simulink library "uplink_4c1r_pd_accu_reg_block"  (Simulink 8.7)
settings: Solver=ode45  StartTime=0.0  StopTime=10.0  RelTol=1e-3
undefined symbols (not defined in the file or in its folder): value
libraries: DSPBAPrim x1, Register x1, DSPBABase x1, Accumulator x1, Peak_Detector x1
settings Model: Creator=bigcat  LastModifiedBy=5g

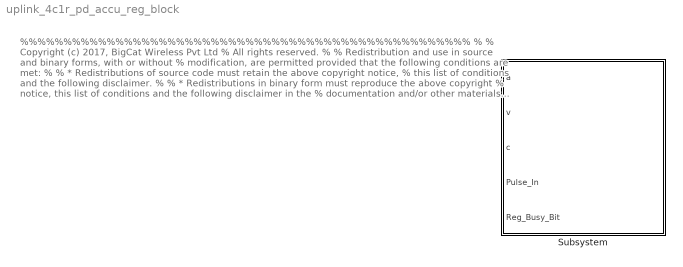
== system uplink_4c1r_pd_accu_reg_block ==
  note: %%%%%%%%%%%%%%%%%%%%%%%%%%%%%%%%%%%%%%%%%%%%%%%%%%%%
      |  %
      |  % Copyright (c) 2017, BigCat Wireless Pvt Ltd
      |  % All rights reserved.
      |  %
      |  % Redistribution and use in source and binary forms, with or without
      |  % modification, are permitted provided that the following conditions are met:
      |  %
      |  %     * Redistributions of source code must retain the above copyright notice,
      |  %       this list of conditions and the following disclaimer.
      |  %
      |  %     * Redistributions in binary form must reproduce the above copyright
      |  %       notice, this list of conditions and the following disclaimer in the
      |  %       documentation and/or other materials provided with the distribution.
      |  %
      |  %     * Neither the name of the copyright holder nor the names of its contributors
      |  %       may be used to endorse or promote products derived from this software
      |  %       without specific prior written permission.
      |  %
      |  %
      |  %
      |  % THIS SOFTWARE IS PROVIDED BY THE COPYRIGHT HOLDERS AND CONTRIBUTORS "AS IS"
      |  % AND ANY EXPRESS OR IMPLIED WARRANTIES, INCLUDING, BUT NOT LIMITED TO, THE
      |  % IMPLIED WARRANTIES OF MERCHANTABILITY AND FITNESS FOR A PARTICULAR PURPOSE ARE
      |  % DISCLAIMED. IN NO EVENT SHALL THE COPYRIGHT HOLDER OR CONTRIBUTORS BE LIABLE
      |  % FOR ANY DIRECT, INDIRECT, INCIDENTAL, SPECIAL, EXEMPLARY, OR CONSEQUENTIAL
      |  % DAMAGES (INCLUDING, BUT NOT LIMITED TO, PROCUREMENT OF SUBSTITUTE GOODS OR
      |  % SERVICES; LOSS OF USE, DATA, OR PROFITS; OR BUSINESS INTERRUPTION) HOWEVER
      |  % CAUSED AND ON ANY THEORY OF LIABILITY, WHETHER IN CONTRACT, STRICT LIABILITY,
      |  % OR TORT (INCLUDING NEGLIGENCE OR OTHERWISE) ARISING IN ANY WAY OUT OF THE USE
      |  % OF THIS SOFTWARE, EVEN IF ADVISED OF THE POSSIBILITY OF SUCH DAMAGE.
      |  %
      |   %%%%%%%%%%%%%%%%%%%%%%%%%%%%%%%%%%%%%%%%%%%%%%%%%%%%%
  Subsystem : Subsystem  mask{Peak_Detector_address=0, Accumulator1_addr=0, Accumulator2_addr=0, Latency=0}
      mask Display:
      | disp('PD_ACCU_REG_BLOCK');
      | port_label('input',1,'d');
      | port_label('input',2,'v');
      | port_label('input',3,'c');
      | port_label('input',4,'pulse_in');
      | port_label('input',5,'Reg_Busy_Bit');

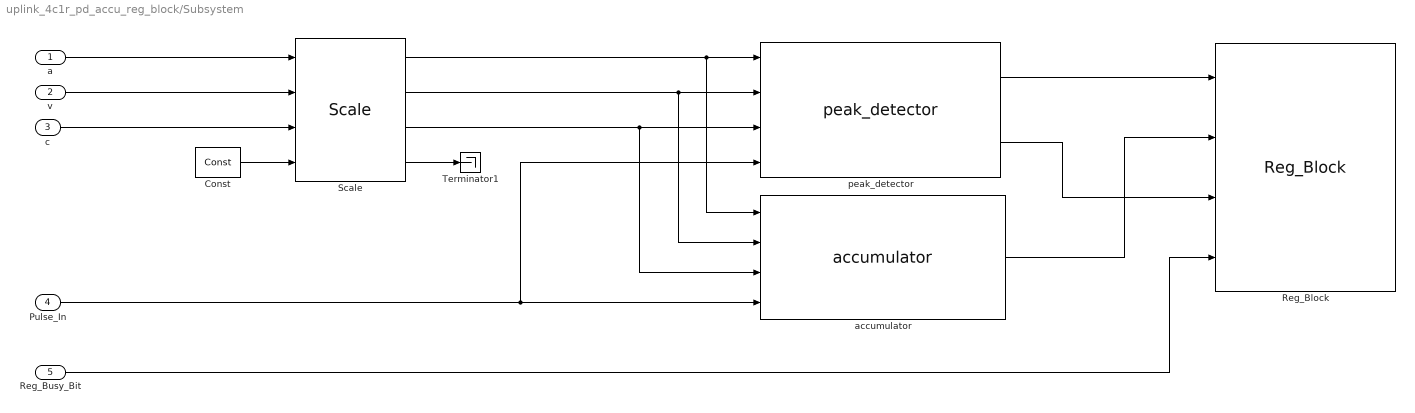
== system uplink_4c1r_pd_accu_reg_block/Subsystem ==
  a : Inport
  v : Inport  Port=2
  c : Inport  Port=3
  Pulse_In : Inport  Port=4
  Reg_Busy_Bit : Inport  Port=5
  Const : DSPBAPrim/Const  primtype=const  nInputs=0  nOutputs=1  omode=Inherit via internal rule  otype=sfix(16)  scale=2^-15  rndmethod=Unbiased  factor=1  satmethod=Symmetric  shift_vec=[0 1 2 -1]  value=0  inPortNames=['+'; '+';]  outPortNames=[' ']  dspbaimage=dspba_prim.jpg  text=fprintf('%s', num2str(value));  style=Optimised  visibilities=8 + 1024  floatPrecision=float32_m23  version=20120820
  Reg_Block : Register/Reg_Block  Peak_Detector_address=Peak_Detector_address  Accumulator1_addr=Accumulator1_addr  Accumulator2_addr=Accumulator2_addr
  Scale : DSPBABase/Scale  otype=sfix(16)  scale=2^-15  rndmethod=Unbiased  factor=1  satmethod=Symmetric  shift_vec=0  latency=6  wideSimulation=off  version=20130807
  Terminator1 : Terminator
  accumulator : Accumulator/accumulator  Latency=Latency
      link override ChannelOut: value=1  packetBeginEnabled=off  latency=21
  peak_detector : Peak_Detector/peak_detector  Latency=Latency
      link override ChannelOut: value=2  packetBeginEnabled=off  latency=21
  wires:
  Scale/3 -> accumulator/3, peak_detector/3
  Const/1 -> Scale/4
  Scale/1 -> accumulator/1, peak_detector/1
  peak_detector/1 -> Reg_Block/1
  a/1 -> Scale/1
  accumulator/1 -> Reg_Block/2
  v/1 -> Scale/2
  Scale/4 -> Terminator1/1
  Scale/2 -> accumulator/2, peak_detector/2
  c/1 -> Scale/3
  Reg_Busy_Bit/1 -> Reg_Block/4
  Pulse_In/1 -> accumulator/4, peak_detector/4
  peak_detector/2 -> Reg_Block/3
